simulink model "SS_design"  (R2025b)
settings: Solver=FixedStepAuto  StartTime=0.0  StopTime=0.0061  FixedStep=1/85e3/1500  RelTol=1e-3
values from neighbouring files (symbols this model uses):
  SS_DB = 0.01    [SS_topology_design.m]
  SS_Duty = 0.5    [SS_topology_design.m]
  SS_Freq = 85e3    (= 85000)    [SS_topology_design.m]
  SS_k = local_get_base_var('SS_k',  0.2)    [SS_find_R_for_power_260407.m]    (also in SS_sweep_R_for_power_260313.m; SS_topology_design.m = 0.2; matlab_workspace.mat = 0.2)
  SS_R = SS_R3    (= 31.23)    [SS_topology_design.m]
  SS_SoftStarting_slope = SS_Vin / SS_SoftStarting_TransientTime    (= 3250000)    [SS_topology_design.m]
  SS_SoftStarting_StartPwmTBCTR = SS_SoftStarting_slope * SS_SoftStarting_StartPwmTime    (= 32.5)    [SS_topology_design.m]
  SS_SoftStarting_StopPwmTBCTR = SS_SoftStarting_slope * SS_SoftStarting_StopPwmTime    (= 19500)    [SS_topology_design.m]
  SS_Vin = local_get_base_var('SS_Vin', 380)    [SS_find_R_for_power_260407.m]    (also in SS_sweep_R_for_power_260313.m; SS_topology_design.m = 650; matlab_workspace.mat = 380)
libraries: fl_lib x26, nesl_utility x25, ee_lib x14, simulink x2
settings Model: Creator=jibin  LastModifiedBy=jibin

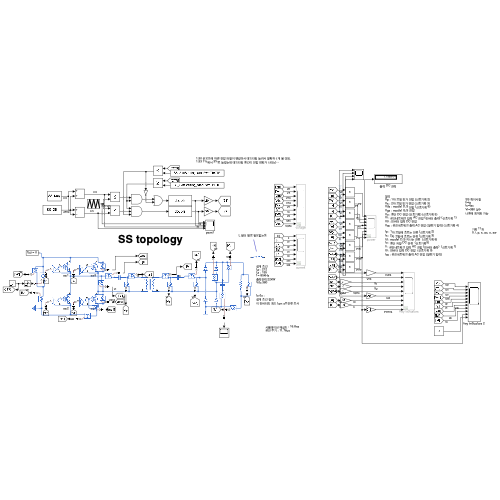
[thumbnail: Simulink's stored preview of the top-level diagram]
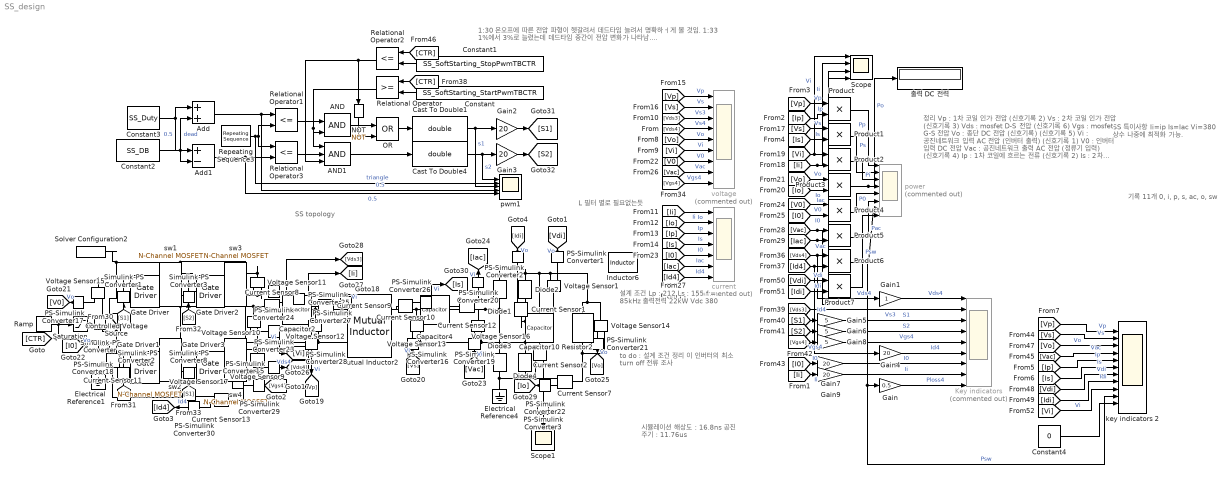
== system SS_design ==
  note: 시뮬레이션 해상도 : 16.8ns
      | 공진 주기 : 11.76us
  note: L 필터 별로 필요없는듯
  note: 기록 11개
      | 0, i, p, s, ac, o, sw
  note: SS 특이사항
      | Ii=ip
      | Is=Iac
      | Vi=380 상수
      | 나중에 최적화 가능.
  note: 정리
      | Vp : 1차 코일 인가 전압 (신호기록 2)
      | Vs : 2차 코일 인가 전압 (신호기록 3)
      | Vds : mosfet D-S 전압 (신호기록 6)
      | Vgs : mosfet G-S 전압
      | Vo : 종단 DC 전압 (신호기록) (신호기록 5)
      | Vi : 공진네트워크 입력 AC 전압 (인버터 출력) (신호기록 1)
      | V0 : 인버터 입력 DC 전압
      | Vac : 공진네트워크 출력 AC 전압 (정류기 입력) (신호기록 4)
      |
      | Ip : 1차 코일에 흐르는 전류 (신호기록 2)
      | Is : 2차 코일에 흐르는 전류 (신호기록 3)
      | Id : mosfet D-S 지나는 전류  (신호기록 6)
      | Io : 종단 저항 DC 전류  (신호기록5)
      | Ii : 공진네트워크 입력 AC 전압 (인버터 출력)  (신호기록 1)
      | I0 : 인버터 입력 DC 전압  (신호기록 0)
      | Iac : 공진네트워크 출력 AC 전압 (정류기 입력)
  note: 설계 조건
      | Lp : 212
      | Ls : 155
      | f = 85kHz
      | 출력전력 22kW
      | Vdc 380
  note: to do :
      | 설계 조건 정리
      | 이 인버터의 최소 turn off 전류 조사
  note: 1:30 온오프에 따른 전압 파형이 헷갈려서 데드타임 늘려서 명확하ㅓ게 볼 것임.
      | 1:33 1%에서 3%로 늘렸는데 데드타임 중간이 전압 변화가 나타남....
  note: SS topology
  AND : Logic  IconShape=distinctive  AllPortsSameDT=off  OutDataTypeStr=boolean
  AND1 : Logic  Inputs=3  IconShape=distinctive  AllPortsSameDT=off  OutDataTypeStr=boolean
  Add : Sum
  Add1 : Sum  Inputs=+-
  Capacitor10 : fl_lib/Electrical/Electrical Elements/Capacitor  c=SS_C_filter F  r=1e-6 Ohm  g=0 1/Ohm  i_specify=off  i_priority=None  i=0 A  i_nominal_specify=off  i_nominal_value=1  i_nominal_unit=A  v_specify=off  v_priority=None  v=0 V  v_nominal_specify=off  v_nominal_value=1  v_nominal_unit=V  vc_specify=off  vc_priority=High  vc=0 V  vc_nominal_specify=off  vc_nominal_value=1  vc_nominal_unit=V
  Capacitor2 : fl_lib/Electrical/Electrical Elements/Capacitor  c=SS_Cp F  r=1e-6 Ohm  g=0 1/Ohm  i_specify=off  i_priority=None  i=0 A  i_nominal_specify=off  i_nominal_value=1  i_nominal_unit=A  v_specify=off  v_priority=None  v=0 V  v_nominal_specify=off  v_nominal_value=1  v_nominal_unit=V  vc_specify=off  vc_priority=High  vc=0 V  vc_nominal_specify=off  vc_nominal_value=1  vc_nominal_unit=V
  Capacitor4 : fl_lib/Electrical/Electrical Elements/Capacitor  c=SS_Cs F  r=1e-6 Ohm  g=0 1/Ohm  i_specify=off  i_priority=None  i=0 A  i_nominal_specify=off  i_nominal_value=1  i_nominal_unit=A  v_specify=off  v_priority=None  v=0 V  v_nominal_specify=off  v_nominal_value=1  v_nominal_unit=V  vc_specify=off  vc_priority=High  vc=0 V  vc_nominal_specify=off  vc_nominal_value=1  vc_nominal_unit=V
  Cast To Double1 : DataTypeConversion  OutDataTypeStr=double  SaturateOnIntegerOverflow=off  RndMeth=Floor
  Cast To Double4 : DataTypeConversion  OutDataTypeStr=double  SaturateOnIntegerOverflow=off  RndMeth=Floor
  Constant : Constant  Value=SS_SoftStarting_StartPwmTBCTR
  Constant1 : Constant  Value=SS_SoftStarting_StopPwmTBCTR
  Constant2 : Constant  Value=SS_DB
  Constant3 : Constant  Value=SS_Duty
  Constant4 : Constant  Value=0
  Controlled Voltage Source : fl_lib/Electrical/Electrical Sources/Controlled Voltage Source
  Current Sensor{1..2,7..13} (9 alike) : fl_lib/Electrical/Electrical Sensors/Current Sensor
  Diode{1..4} (4 alike) : ee_lib/Semiconductors & Converters/Diode  ModelType=ee.enum.diode.modelType.pwl  TableType=ee.enum.diode.tableType.IfMat  IfMat=[.07, .12, .19, 1.75, 4.24, 7.32, 11.2; .16, .3, .72, 2.14, 5.02, 8.35, 13.12] A  VfMat=[.9, 1.15, 1.25, 1.5, 1.75, 2.17, 2.6, 2.85; .58, .68, .75, 1.1, 1.38, 1.77, 2.27, 2.7] V  TjVec=[25, 125] degC  VfVec=[.5, .7, .9, 1.3, 1.7, 2.1, 2.5] V  IfVec=[.1, .2, .5, 1, 2, 4, 7, 10] A  IrMat=[1e-06, 2e-06, 5e-06, 1e-05, 2.5e-05, 5e-05, .0001; 2e-06, 5e-06, 1e-05, 4e-05, 8e-05, .0002, .0005] A  VrMat=[10, 100, 200, 250, 300, 325, 350; 10, 70, 160, 220, 270, 300, 320] V  VrVec=[10, 20, 40, 50, 70, 80, 100] V  IrVec=[1e-06, 2e-06, 5e-06, 1e-05, 2e-05, 5e-05, .0001] A  Vf=1 V  Ron=0.02 Ohm  Goff=1e-8 S  prmExp=ee.enum.diode.expParam.useTwo  I12=[.0137, .545] A  V12=[.6, .7] V  RS=0 Ohm  Tmeas=298.15 K  IS=1e-12 A  ec=1  I1=0.0137 A  V1=0.6 V  N_series=1  N_parallel=2  ZenerEnable=false  Rz=0.3 Ohm  BV=inf V  C_param=ee.enum.diode.capParam.fixed  CJ=0 pF  CJ0=5 pF  Vvec=[.1, 10, 100] V  Cvec=[3.5, 1, .4] pF  VJ=1 V  Mgrad=0.5  FC=0.5  Q_param=ee.enum.diode.recoveryParam.off  iRM=-7.15 A  iF=4 A  didt=-750 A/us  trr_factor=3  trr=115 ns  Qrr=150 nA*s  Vr=-600 V  Ls=150 nH  Erec=0.03 J  TT=50 ns  tau=100 ns  T_param=ee.enum.diode.temperatureParam.off  Tdevice=298.15 K  I1_T2=0.245 A  V1_T2=0.5 V  IS_T2=1.25e-7 A  Tmeas2=125 degC  XTI_param=ee.enum.diode.xtiParam.pn  XTI=3  EG_param=ee.enum.diode.egapParam.material_si  EG=1.11 eV  dBVdT=0 V/K  enable_fault_input=simscape.enum.onoff.off  i_specify=off  i_priority=None  i=0 A  i_nominal_specify=off  i_nominal_value=1  i_nominal_unit=A  v_specify=off  v_priority=None  v=0 V  v_nominal_specify=off  v_nominal_value=1  v_nominal_unit=V  v_capacitor_specify=off  v_capacitor_priority=None  v_capacitor=0 V  v_capacitor_nominal_specify=off  v_capacitor_nominal_value=1  v_capacitor_nominal_unit=V  Qj_specify=off  Qj_priority=High  Qj=0 C  Qj_nominal_specify=off  Qj_nominal_value=1  Qj_nominal_unit=C  i_diode_specify=off  i_diode_priority=None  i_diode=0 A  i_diode_nominal_specify=off  i_diode_nominal_value=1  i_diode_nominal_unit=A  v_diode_specify=off  v_diode_priority=None  v_diode=0 V  v_diode_nominal_specify=off  v_diode_nominal_value=1  v_diode_nominal_unit=V  i_capacitor_specify=off  i_capacitor_priority=None  i_capacitor=0 A  i_capacitor_nominal_specify=off  i_capacitor_nominal_value=1  i_capacitor_nominal_unit=A  power_dissipated_specify=off  power_dissipated_priority=None  power_dissipated=0 W  power_dissipated_nominal_specify=off  power_dissipated_nominal_value=1  power_dissipated_nominal_unit=W  fidelity_level=ee.enum.diode.fidelity.includeChargeDyn  rec_loss_model=ee.enum.diode.reverseRecoveryModel.fixed  ErecVal=0 J  scaleWithIandV=true  ErecMat=zeros(2, 3) J  TjrecVec=[298.15, 398.15] K  IfrecVec=[.1, 1, 10] A  IrecVal=10 A  VrecVal=10 V  tFilter=1 / 1000 / 100 s  thermal_network_parameterization=ee.enum.thermalNetworkTopology.junctionCase  Rth=[0, 10] K/W  Rth_Cauer=[1, 3, 10] K/W  Rth_Foster=[.08, .14, .22, .16] K/W  thermal_mass_parameterization=ee.enum.thermalNetwork.timeconstant  thermal_mass=[0, 1] J/K  thermal_mass_Cauer=[.1, .3, 1] J/K  thermal_mass_Foster=[.001, .005, .05, .5] J/K  thermal_time_constant=[0, 10] s  thermal_time_constant_Cauer=[1, 3, 10] s  thermal_time_constant_Foster=[7e-05, .0007, .01, .08] s  thermal_mass_initial_temperatures=[25, 25] degC  thermal_mass_initial_temperatures_Cauer=[25, 25, 25] degC  junction_thermal_mass=0.01 J/K  Tvec_initial_Foster=[25, 25, 25, 25] degC  no_thermal_network=0  junction_temperature_specify=off  junction_temperature_priority=None  junction_temperature=25 degC  junction_temperature_nominal_specify=off  junction_temperature_nominal_value=1  junction_temperature_nominal_unit=degC
  Electrical Reference1 : fl_lib/Electrical/Electrical Elements/Electrical Reference
  Electrical Reference4 : fl_lib/Electrical/Electrical Elements/Electrical Reference
  Gain : Gain  Gain=0.5
  Gain1 : Gain
  Gain{2..4,7,9} (5 alike) : Gain  Gain=20
  Gain5 : Gain  Gain=5
  Gain6 : Gain  Gain=5
  Gain8 : Gain  Gain=5
  Gate Driver{,1..3} (4 alike) : ee_lib/Semiconductors & Converters/Gate Driver  port_option=ee.enum.controlport.ps  uHigh=2.0 V  uLow=0.8 V  uHighValue=0.7  uLowValue=0.3  vHigh=SS_driv_Von V  vLow=SS_driv_Voff V  tHigh=0 ns  tLow=0 ns  parameterization=ee.enum.semiconductors.gateDriverParam.outputImpedance  rHigh=15 Ohm  rLow=15 Ohm  tRise=20 ns  tFall=20 ns  cLoad=10 nF  ZonTime_specify=off  ZonTime_priority=None  ZonTime=0 s  ZoffTime_specify=off  ZoffTime_priority=None  ZoffTime=0 s
      settings: InternalSimscapePortConfiguration="{\"Bottom\":[],\"Left\":[{\"id\":\"u\",\"label\":\"u\",\"type\":\"input\"}],\"Right\":[{\"id\":\"G\",\"label\":\"G\",\"type\":\"foundation.electrical.electrical\"},{\"id\":\"S\",\"label\":\"S\",\"type\":\"foundation.electrical.electrical\"}],\"Top\":[]}"
  Inductor6 : ee_lib/Passive/Inductor  l=SS_L_filter H  enable_L_tol=ee.enum.toleranceApplication.none  L_tol=20  tol_distribution=ee.enum.toleranceDistribution.uniform  nSigma=4  r=0 Ohm  g=1e-9 1/Ohm  enable_operating_limits=ee.enum.enable.no  operating_limit_action=ee.enum.passive.reportOpLim.warn  max_working_current=1 A  power_rating=1 W  i_L_specify=off  i_L_priority=High  i_L=0 A  i_L_nominal_specify=off  i_L_nominal_value=1  i_L_nominal_unit=A
  Key indicators : Scope  Commented=on  NumInputPorts=9
      settings: ActiveDisplayYMinimum=-3153.8043983257576  ActiveDisplayYMaximum=2006.1519840284409  DataLoggingVariableName=ScopeData3
  Mutual Inductor2 : ee_lib/Passive/Transformers/Mutual Inductor  L1=SS_Lp H  L2=SS_Ls H  k=SS_k  L_tol=0  enable_L1_tol=ee.enum.toleranceApplication.none  L1_tol_distribution=ee.enum.toleranceDistribution.uniform  L1_nSigma=4  enable_L2_tol=ee.enum.toleranceApplication.none  L2_tol_distribution=ee.enum.toleranceDistribution.uniform  L2_nSigma=4  r=[.001, .001] Ohm  g=[1e-09, 1e-09] 1/Ohm  enable_operating_limits=ee.enum.enable.no  operating_limit_action=ee.enum.passive.reportOpLim.warn  max_working_current=1 A  power_rating=1 W  iL1_specify=off  iL1_priority=High  iL1=0 A  iL1_nominal_specify=off  iL1_nominal_value=1  iL1_nominal_unit=A  iL2_specify=off  iL2_priority=High  iL2=0 A  iL2_nominal_specify=off  iL2_nominal_value=1  iL2_nominal_unit=A
      settings: InternalSimscapePortConfiguration="{\"Bottom\":[],\"Left\":[{\"id\":\"p1\",\"label\":\"1+\",\"type\":\"foundation.electrical.electrical\"},{\"id\":\"n1\",\"label\":\"1-\",\"type\":\"foundation.electrical.electrical\"}],\"Right\":[{\"id\":\"p2\",\"label\":\"2+\",\"type\":\"foundation.electrical.electrical\"},{\"id\":\"n2\",\"label\":\"2-\",\"type\":\"foundation.electrical.electrical\"}],\"Top\":[]}"
  NOT : Logic  Operator=NOT  IconShape=distinctive  AllPortsSameDT=off  OutDataTypeStr=boolean
  OR : Logic  Operator=OR  IconShape=distinctive  AllPortsSameDT=off  OutDataTypeStr=boolean
  PS-Simulink Converter{1..3,15..30} (19 alike) : nesl_utility/PS-Simulink Converter  PhysicalDomain=network_engine_domain  SubClassName=ps_output  LeftPortType=input  RightPortType=output  PseudoPeriodic=off  Frequencies=[]  VectorFormat=inherit  Unit=inherit  AffineConversion=off
  Product{,1..7} (8 alike) : Product
  Ramp : simulink/Sources/Ramp  slope=SS_SoftStarting_slope  start=SS_SoftStarting_delayed  InitialOutput=0
  Relational Operator : RelationalOperator  OutDataTypeStr=boolean  RndMeth=Simplest  InputSameDT=off
  Relational Operator1 : RelationalOperator  Operator=<=  OutDataTypeStr=boolean  RndMeth=Simplest  InputSameDT=off
  Relational Operator2 : RelationalOperator  Operator=<=  OutDataTypeStr=boolean  RndMeth=Simplest  InputSameDT=off
  Relational Operator3 : RelationalOperator  Operator=<=  OutDataTypeStr=boolean  RndMeth=Simplest  InputSameDT=off
  Repeating Sequence3 : simulink/Sources/Repeating Sequence  rep_seq_t=[0 1/SS_Freq/2 1/SS_Freq]  rep_seq_y=[0 1 0]
  Resistor2 : fl_lib/Electrical/Electrical Elements/Resistor  R=SS_R Ohm  i_specify=off  i_priority=None  i=0 A  i_nominal_specify=off  i_nominal_value=1  i_nominal_unit=A  v_specify=off  v_priority=None  v=0 V  v_nominal_specify=off  v_nominal_value=1  v_nominal_unit=V
  Saturation : Saturate  UpperLimit=SS_Vin  LowerLimit=0
  Scope : Scope  NumInputPorts=4
      settings: ActiveDisplayYMinimum=-209.64709270846973  ActiveDisplayYMaximum=229.34788450491459  DataLoggingVariableName=ScopeData6
  Scope1 : Scope
      settings: ActiveDisplayYMinimum=-22.784253900925922  ActiveDisplayYMaximum=48.876040057618852  DataLoggingVariableName=ScopeData7
  Simulink-PS Converter{,1..3,8} (5 alike) : nesl_utility/Simulink-PS Converter  PhysicalDomain=network_engine_domain  SubClassName=ps_input  LeftPortType=input  RightPortType=output  PseudoPeriodic=off  Frequencies=[]  NoiseDistribution=none  NoiseParameters=[]  Unit=1  AffineConversion=off  FilteringAndDerivatives=provide  SimscapeFilterOrder=1  InputFilterTimeConstant=0.001  UdotUserProvided=0
  Solver Configuration2 : nesl_utility/Solver Configuration  PhysicalDomain=network_engine_domain  SubClassName=solver  LeftPortType=input  RightPortType=generic  Tones=[]  Harmonics=[]  SimulateNoise=off  Profile=off  UseLocalSampling=off  EnableSwitchedLinearOptims=on  FrequencyDomain=off  UseCCode=off  RelTol=0.001  AbsTol=0.001  MinStep=1e-09  ToWorkspace=off  RevertToSquareIcSolve=off  NumHomotopyIterations=100  PhasorMode=off  PhasorModeNumHarmonics=1  ConsistencySolver=NEWTON_XTOL_AFTER_FTOL  IndexReductionMethod=DerivativeReplacement  DoDC=off  ResidualTolerance=1e-09  ConsistencyTolSource=LOCAL  ConsistencyAbsTol=0.001  ConsistencyRelTol=0.001  ConsistencyTolFactor=0.001  UseLocalSolver=on  LocalSolverChoice=NE_BACKWARD_EULER_ADVANCER  ResolveIndetEquations=on  FunctionEvalNumThread=1  LocalSolverSampleTime=1/85e3/1500  DoFixedCost=off  MaxNonlinIter=3  MaxModeIter=2  ComputeImpulses=off  ImpulseIterations=2  LinearAlgebra=auto  LinearAlgebraNumThread=0  EquationFormulation=NE_TIME_EF  DelaysMemoryBudget=1024  AutomaticFiltering=on  FilteringTimeConstant=0.001  PartitionStorageMethod=AS_NEEDED  PartitionMemoryBudget=1024  PartitionMethod=ROBUST  MultibodyUseLocalSolver=off  MultibodyLocalSolverChoice=ODE1  MultibodyLocalSolverSampleTime=0.001
  Voltage Sensor{1,9..17} (10 alike) : fl_lib/Electrical/Electrical Sensors/Voltage Sensor
  current : Scope  Commented=on  NumInputPorts=7
      settings: ActiveDisplayYMinimum=-15.036920895804315  ActiveDisplayYMaximum=15.036548168459881  DataLoggingVariableName=ScopeData5
  key indicators 2 : Scope  NumInputPorts=11
      settings: ActiveDisplayYMinimum=-48.81005828333268  ActiveDisplayYMaximum=48.809899474226675  DataLoggingVariableName=ScopeData4
  power : Scope  Commented=on  NumInputPorts=8
      settings: ActiveDisplayYMinimum=-2917.4741036570072  ActiveDisplayYMaximum=7376.975692043733
  pwm1 : Scope  NumInputPorts=5
      settings: ActiveDisplayYMinimum=-0.12497287522603978  ActiveDisplayYMaximum=1.1247558770343582
  sw{1..4} (4 alike) : ee_lib/Semiconductors & Converters/N-Channel MOSFET  paramTerminal=ee.enum.mosfet.numberOfTerminals.three  parameterization=ee.enum.mosfet.parameterization.datasheet  Beta=5.0 A/V^2  Rds=15 mOhm  Id=100 A  Vgs=15 V  Vth=2.5 V  Vth0=1.7 V  lam=0 1/V  gamma_vth=0.5 V^(1/2)  phib=0.5 V  Vth1=1.9071 V  Vbs1=-1 V  Vth2=2.066 V  Vbs2=-2 V  Tmeas=25 degC  Vgs_vec=[-1, -.5, 2, 3, 4, 5] V  Vds_vec=[0, 2, 4, 8, 12, 16, 20] V  Vbs_vec=[0, -4, -6, -12] V  T_vec=[25, 125] degC  Vth_vec=[.4, 1.2, 1.4, 1.45] V  Vth_mat=[.4, .35; 1.2, 1.15; 1.4, 1.35; 1.45, 1.4] V  Ids_mat=[0, 0, 0, 0, 0, 0, 0; 0, 0, 0, 0, 0, 0, 0; 0, .003, .0038, .0043, .0046, .0048, .0049; 0, .0055, .008, .009, .0095, .01, .0101; 0, .0115, .016, .018, .019, .0195, .02; 0, .0152, .0225, .0265, .028, .0295, .03] A  Ids_mat0=[0, 0, 0, 0, 0, 0, 0; 0, 0, 0, 0, 0, 0, 0; 0, .003, .0038, .0043, .0046, .0048, .0049; 0, .0055, .008, .009, .0095, .01, .0101; 0, .0115, .016, .018, .019, .0195, .02; 0, .0152, .0225, .0265, .028, .0295, .03] A  Ids_mat_3D=zeros(6, 7, 2) A  Ids_mat_3D0=zeros(6, 7, 2) A  IV_table_symmetry=ee.enum.mosfet.symmetricNIV.no  RS=0.0001 Ohm  RD=0.01 Ohm  RB=0.001 Ohm  LeadRs=1e-4 Ohm  LeadRd=1e-4 Ohm  LeadRg=1e-4 Ohm  LeadRb=0 Ohm  LS=1e-4 nH  LD=1e-4 nH  LG=1e-4 nH  LB=0 nH  C_param=ee.enum.mosfet.capacitanceParam.fixedciss  C_GS=270 pF  C_GD=80 pF  C_GB=0 pF  C_DS=0 pF  C_iss=SS_MSFT_Ciss F  C_rss=SS_MSFT_Crss F  C_oss=SS_MSFT_Coss F  C_iss_vec=[720, 700, 590, 470, 390, 310] pF  C_rss_vec=[450, 400, 300, 190, 95, 55] pF  C_oss_vec=[900, 810, 690, 420, 270, 170] pF  C_GS_vec=[270, 300, 290, 280, 295, 255] pF  C_GD_vec=[450, 400, 300, 190, 95, 55] pF  C_GB_vec=[270, 300, 290, 280, 295, 255] pF  C_Vgs_vec=0 V  C_DS_vec=[450, 410, 390, 230, 175, 115] pF  C_Vds_vec=[.1, .3, 1, 3, 10, 30] V  V_GS_for_cap_data=0 V  charge_linearity_param=ee.enum.mosfet.cgdLinearity.constant  C_OX=200 pF  V_C_OX=-0.5 V  charge_linearity_param_vgb=ee.enum.mosfet.cgbLinearity.instantly  charge_linearity_param_with_vgb=ee.enum.mosfet.cgbLinearityWithSeparateCgb.instantly  Di_param=ee.enum.mosfet.diodeParam.exponential  IsDiode=1e-12 A  Vbi=0.6 V  n=1  Cj0Diode=0 pF  TT=150e-9 s  Tmeas_dio=25 degC  TableTypeNoT=ee.enum.mosfet.tableType.IfMat  TableType=ee.enum.diode.tableType.IfMat  IfVec=[.07, .12, .19, 1.75, 4.24, 7.32, 11.2] A  IfMat=[.07, .12, .19, 1.75, 4.24, 7.32, 11.2; .16, .3, .72, 2.14, 4.02, 6.35, 9.12] A  VfVecV=[.9, 1.15, 1.25, 1.5, 1.75, 2.17, 2.6, 2.85] V  VfMatV=[.9, 1.15, 1.25, 1.5, 1.75, 2.17, 2.6, 2.85; .58, .68, .75, 1.1, 1.38, 1.77, 2.27, 2.7] V  TjVec=[25, 125] degC  VfVec=[.5, .7, .9, 1.3, 1.7, 2.1, 2.5] V  IfVecV=[.1, .2, .5, 1, 2, 4, 7, 10] A  diode_Goff=1e-12 1/Ohm  prmDatasheet=ee.enum.temperatureParameterization.none  prmEquCoeff=ee.enum.temperatureParameterization.none  dVth_dT=-6 mV/K  dVth0_dT=-6 mV/K  Rds_T2=0.037 Ohm  BEXDatasheet=-1.5  BEXEquCoeff=-1.5  etaisDatasheet=3  etaisEquCoeff=3  Tmeas2=125 degC  etaisTabulated=3  TdeviceDatasheet=25 degC  TdeviceEquCoeff=25 degC  TdeviceTabulated=25 degC  i_g_specify=off  i_g_priority=None  i_g=0 A  i_g_nominal_specify=off  i_g_nominal_value=1  i_g_nominal_unit=A  i_d_specify=off  i_d_priority=None  i_d=0 A  i_d_nominal_specify=off  i_d_nominal_value=1  i_d_nominal_unit=A  i_b_specify=off  i_b_priority=None  i_b=0 A  i_b_nominal_specify=off  i_b_nominal_value=1  i_b_nominal_unit=A  voltage_gs_specify=off  voltage_gs_priority=None  voltage_gs=0 V  voltage_gs_nominal_specify=off  voltage_gs_nominal_value=1  voltage_gs_nominal_unit=V  voltage_ds_specify=off  voltage_ds_priority=None  voltage_ds=0 V  voltage_ds_nominal_specify=off  voltage_ds_nominal_value=1  voltage_ds_nominal_unit=V  voltage_bs_specify=off  voltage_bs_priority=None  voltage_bs=0 V  voltage_bs_nominal_specify=off  voltage_bs_nominal_value=1  voltage_bs_nominal_unit=V  v_Cgs_specify=on  v_Cgs_priority=None  v_Cgs=0 V  v_Cgs_nominal_specify=off  v_Cgs_nominal_value=1  v_Cgs_nominal_unit=V  v_Cds_specify=on  v_Cds_priority=None  v_Cds=0 V  v_Cds_nominal_specify=off  v_Cds_nominal_value=1  v_Cds_nominal_unit=V  v_Cbs_specify=off  v_Cbs_priority=High  v_Cbs=0 V  v_Cbs_nominal_specify=off  v_Cbs_nominal_value=1  v_Cbs_nominal_unit=V  thermal_network_parameterization=ee.enum.thermalNetworkTopology.junctionCase  Rth=[0, 10] K/W  Rth_Cauer=[1, 3, 10] K/W  Rth_Foster=[.08, .14, .22, .16] K/W  thermal_mass_parameterization=ee.enum.thermalNetwork.timeconstant  thermal_mass=[0, 1] J/K  thermal_mass_Cauer=[.1, .3, 1] J/K  thermal_mass_Foster=[.001, .005, .05, .5] J/K  thermal_time_constant=[0, 10] s  thermal_time_constant_Cauer=[1, 3, 10] s  thermal_time_constant_Foster=[7e-05, .0007, .01, .08] s  thermal_mass_initial_temperatures=[25, 25] degC  thermal_mass_initial_temperatures_Cauer=[25, 25, 25] degC  Tvec_initial_Foster=[25, 25, 25, 25] degC  betaref=18 A/V^2  Vfbref=-1.1 V  gamma=3.5 V^(1/2)  phib2ref=1 V  thesatref=0.4 1/V  alpha=0  Vp=5e-2 V  thesrref=0 1/V  m=8  Tref=25 degC  Rsref=2e-3 Ohm  Rdref=0.17 Ohm  Rgref=8.4 Ohm  Rbref=2e-3 Ohm  Cox=1500 pF  Cgso=100 pF  Cgdo=14 pF  Isref=5.2e-13 A  Cj0=480 pF  Tprm=1  etabet=1.3  Stvfb=5e-4 V/K  Stphib=-8.5e-4 V/K  etasat=1.04  etasr=0.65  etar=0.95  etais=3  Tsim=25 degC  Ig_specify=off  Ig_priority=None  Ig=0 A  Ig_nominal_specify=off  Ig_nominal_value=1  Ig_nominal_unit=nA  Ids_specify=off  Ids_priority=None  Ids=0 A  Ids_nominal_specify=off  Ids_nominal_value=1  Ids_nominal_unit=A  Ib_specify=off  Ib_priority=None  Ib=0 A  Ib_nominal_specify=off  Ib_nominal_value=1  Ib_nominal_unit=uA  V_gs_specify=off  V_gs_priority=None  V_gs=0 V  V_gs_nominal_specify=off  V_gs_nominal_value=1  V_gs_nominal_unit=V  V_ds_specify=off  V_ds_priority=None  V_ds=0 V  V_ds_nominal_specify=off  V_ds_nominal_value=1  V_ds_nominal_unit=V  V_bs_specify=off  V_bs_priority=None  V_bs=0 V  V_bs_nominal_specify=off  V_bs_nominal_value=1  V_bs_nominal_unit=V  QGoverCox_specify=off  QGoverCox_priority=None  QGoverCox=0 V  QGoverCox_nominal_specify=off  QGoverCox_nominal_value=1  QGoverCox_nominal_unit=V  QDoverCox_specify=off  QDoverCox_priority=None  QDoverCox=0 V  QDoverCox_nominal_specify=off  QDoverCox_nominal_value=1  QDoverCox_nominal_unit=V  QBoverCox_specify=off  QBoverCox_priority=None  QBoverCox=0 V  QBoverCox_nominal_specify=off  QBoverCox_nominal_value=1  QBoverCox_nominal_unit=V  T0=[25, 25] degC  T0_Cauer=[25, 25, 25] degC
  voltage : Scope  Commented=on  NumInputPorts=9
      settings: ActiveDisplayYMinimum=-88.829095611503391  ActiveDisplayYMaximum=432.28140472052308  DataLoggingVariableName=ScopeData2
  출력 DC 전력 : Display
  wires:
  Product6/1 -> key indicators 2/10, Gain/1, power/7  "Psw"
  Add1/1 -> pwm1/5, Relational Operator3/2  "0.5"
  [Vds4] -> voltage/4  "Vs4"
  [Io] -> current/2  "Io"
  Product4/1 -> power/5  "P0"
  Product/1 -> power/1  "Pp"
  [I0] -> current/5  "I0"
  Relational Operator3/1 -> AND1/2
  Gain5/1 -> Key indicators/3  "S1"
  PS-Simulink Converter25/1 -> [Ii]
  OR/1 -> Cast To Double1/1
  [Ii] -> Scope/2, Product2/2  "Ii"
  [Vi] -> voltage/6  "Vi"
  PS-Simulink Converter29/1 -> [Vgs4]
  PS-Simulink Converter26/1 -> [Is]  "Vi"
  [Iac] -> Scope/4, Product5/2  "Iac"
  [S2] -> Simulink-PS Converter3/1
  Product2/1 -> power/3  "Pi"
  Gain1/1 -> Key indicators/1  "Vds4"
  [S1] -> Simulink-PS Converter1/1
  Relational Operator1/1 -> AND/1
  [CTR] -> Relational Operator2/1
  [Vi] -> Scope/1, Product2/1  "Vi"
  AND/1 -> OR/1
  Constant2/1 -> Add/2, Add1/2  "dead"
  Cast To Double1/1 -> Gain2/1, pwm1/3  "s1"
  [CTR] -> Relational Operator/1
  [Ip] -> current/3  "Ip"
  [Ip] -> Product/2  "Ip"
  NOT/1 -> OR/2
  [Vs] -> Product1/1  "Vs"
  Gain8/1 -> Key indicators/5  "Vgs4"
  [Id4] -> Gain4/1, Product6/2  "Id4"
  Relational Operator/1 -> AND1/1, AND/2
  Product5/1 -> power/6  "Pac"
  Constant3/1 -> Add/1, Add1/1  "0.5"
  [V0] -> Product4/1  "V0"
  Cast To Double4/1 -> Gain3/1, pwm1/1  "s2"
  Gain2/1 -> [S1]
  [Vo] -> voltage/5  "Vo"
  [Vac] -> voltage/8  "Vac"
  [S1] -> Simulink-PS Converter8/1
  [Io] -> Product3/2  "Io"
  Gain4/1 -> Key indicators/6  "Id4"
  PS-Simulink Converter19/1 -> [Vac]  "Vi"
  PS-Simulink Converter30/1 -> [Id4]  "Id4"
  [Id4] -> current/7  "Id4"
  [Vgs4] -> Gain8/1  "Vgs4"
  [S2] -> Simulink-PS Converter2/1
  [Vo] -> Product3/1  "Vo"
  PS-Simulink Converter21/1 -> [Vo]  "Vo"
  PS-Simulink Converter17/1 -> [V0]  "Vo"
  Repeating Sequence3/1 -> pwm1/2, Relational Operator1/2, Relational Operator3/1  "triangle"
  [S2] -> Gain6/1
  [Vac] -> Scope/3, Product5/1  "Vac"
  PS-Simulink Converter22/1 -> [Io]
  Gain6/1 -> Key indicators/4  "S2"
  Saturation/1 -> Simulink-PS Converter/1
  PS-Simulink Converter18/1 -> [I0]  "Vo"
  Product1/1 -> power/2  "Ps"
  Ramp/1 -> Saturation/1, [CTR]
  [Vp] -> Product/1  "Vp"
  PS-Simulink Converter27/1 -> [Ip]  "Vi"
  [Vds3] -> Key indicators/2  "Vs3"
  Gain3/1 -> [S2]
  Gain7/1 -> Key indicators/7  "I0"
  PS-Simulink Converter16/1 -> [Vs]  "Vi"
  [Vds3] -> voltage/3  "Vs3"
  AND1/1 -> Cast To Double4/1
  PS-Simulink Converter20/1 -> [Iac]  "Vi"
  Constant/1 -> Relational Operator/2
  PS-Simulink Converter24/1 -> [Vds3]
  [Vgs4] -> voltage/9  "Vgs4"
  [I0] -> Product4/2  "I0"
  Product3/1 -> 출력 DC 전력/1, power/4  "Po"
  PS-Simulink Converter28/1 -> [Vp]  "Vi"
  [Is] -> Product1/2  "Is"
  [S1] -> Gain5/1
  [Ii] -> current/1  "Ii"
  [V0] -> voltage/7  "V0"
  [I0] -> Gain7/1  "I0"
  [Vs] -> voltage/2  "Vs"
  Relational Operator2/1 -> NOT/1, AND1/3
  [Iac] -> current/6  "Iac"
  Gain/1 -> Key indicators/9  "Ploss4"
  [Vp] -> voltage/1  "Vp"
  Constant1/1 -> Relational Operator2/2
  PS-Simulink Converter23/1 -> [Vi]  "Vi"
  [Vds4] -> Gain1/1, Product6/1  "Vds4"
  PS-Simulink Converter15/1 -> [Vds4]  "Vds4"
  Add/1 -> pwm1/4, Relational Operator1/1  "0.5"
  [Is] -> current/4  "Is"
  [Ii] -> Gain9/1  "Ii"
  Gain9/1 -> Key indicators/8  "Ii"
  [Vp] -> key indicators 2/1  "Vp"
  [Vs] -> key indicators 2/2  "Vs"
  [Vo] -> key indicators 2/3  "Vo"
  [Vac] -> key indicators 2/4  "Vac"
  [Ip] -> key indicators 2/5  "Ip"
  [Is] -> key indicators 2/6  "Is"
  PS-Simulink Converter1/1 -> [Vdi]  "Vo"
  [Vdi] -> key indicators 2/7  "Vdi"
  [Idi] -> key indicators 2/8  "Idi"
  PS-Simulink Converter2/1 -> [Idi]  "Vo"
  [Vdi] -> Product7/1  "Vdi"
  [Idi] -> Product7/2  "Idi"
  Product7/1 -> power/8  "Psw"
  [Vi] -> key indicators 2/9  "Vi"
  Constant4/1 -> key indicators 2/11
  PS-Simulink Converter3/1 -> Scope1/1
  connections:
  Voltage Sensor10/RConn2 -- Voltage Sensor12/RConn2 -- Mutual Inductor2/LConn2 -- Voltage Sensor9/LConn1 -- sw4/RConn1 -- Voltage Sensor11/RConn2 -- sw3/RConn2 -- Gate Driver2/RConn2
  Diode4/LConn1 -- Diode3/LConn1 -- Electrical Reference4/LConn1 -- Current Sensor2/RConn2 -- Current Sensor7/RConn2
  Gate Driver/RConn2 -- sw1/RConn2 -- Current Sensor8/LConn1 -- Voltage Sensor10/LConn1 -- sw2/RConn1
  Gate Driver3/RConn1 -- sw4/LConn1 -- Voltage Sensor17/LConn1
  Gate Driver3/RConn2 -- Voltage Sensor9/RConn2 -- sw4/RConn2 -- Current Sensor13/LConn1 -- Voltage Sensor17/RConn2
  Voltage Sensor15/RConn2 -- Current Sensor11/RConn2 -- Controlled Voltage Source/RConn2
  sw2/RConn2 -- Gate Driver1/RConn2 -- Electrical Reference1/LConn1 -- Current Sensor11/LConn1 -- Current Sensor13/RConn2
  Resistor2/RConn1 -- Current Sensor7/LConn1 -- Voltage Sensor14/RConn2
  sw1/RConn1 -- Controlled Voltage Source/LConn1 -- Voltage Sensor15/LConn1 -- Solver Configuration2/RConn1 -- Voltage Sensor11/LConn1 -- sw3/RConn1
  Capacitor10/LConn1 -- Diode2/RConn1 -- Diode1/RConn1 -- Resistor2/LConn1 -- Voltage Sensor14/LConn1 -- Voltage Sensor1/RConn2
  Mutual Inductor2/RConn2 -- Diode4/RConn1 -- Current Sensor1/LConn1 -- Voltage Sensor1/LConn1 -- Voltage Sensor16/RConn2 -- Voltage Sensor13/RConn2
  Capacitor2/RConn1 -- Current Sensor9/LConn1 -- Voltage Sensor12/LConn1
  Capacitor4/LConn1 -- Voltage Sensor13/LConn1 -- Current Sensor10/RConn2
  Current Sensor12/RConn2 -- Voltage Sensor16/LConn1 -- Diode3/RConn1 -- Diode1/LConn1
  PS-Simulink Converter17/LConn1 -- Voltage Sensor15/RConn1
  PS-Simulink Converter27/LConn1 -- Current Sensor9/RConn1
  Voltage Sensor16/RConn1 -- PS-Simulink Converter19/LConn1
  Current Sensor7/RConn1 -- PS-Simulink Converter22/LConn1
  Simulink-PS Converter2/RConn1 -- Gate Driver1/LConn1
  Gate Driver3/LConn1 -- Simulink-PS Converter8/RConn1
  Simulink-PS Converter1/RConn1 -- Gate Driver/LConn1
  PS-Simulink Converter20/LConn1 -- Current Sensor12/RConn1
  sw3/LConn1 -- Gate Driver2/RConn1
  PS-Simulink Converter21/LConn1 -- Voltage Sensor14/RConn1
  Current Sensor13/RConn1 -- PS-Simulink Converter30/LConn1
  Gate Driver1/RConn1 -- sw2/LConn1
  Simulink-PS Converter3/RConn1 -- Gate Driver2/LConn1
  PS-Simulink Converter18/LConn1 -- Current Sensor11/RConn1
  Current Sensor9/RConn2 -- Mutual Inductor2/LConn1
  PS-Simulink Converter25/LConn1 -- Current Sensor8/RConn1
  Mutual Inductor2/RConn1 -- Current Sensor10/LConn1
  Capacitor2/LConn1 -- Current Sensor8/RConn2
  Voltage Sensor12/RConn1 -- PS-Simulink Converter28/LConn1
  Voltage Sensor13/RConn1 -- PS-Simulink Converter16/LConn1
  PS-Simulink Converter24/LConn1 -- Voltage Sensor11/RConn1
  PS-Simulink Converter15/LConn1 -- Voltage Sensor9/RConn1
  PS-Simulink Converter29/LConn1 -- Voltage Sensor17/RConn1
  sw1/LConn1 -- Gate Driver/RConn1
  Simulink-PS Converter/RConn1 -- Controlled Voltage Source/RConn1
  PS-Simulink Converter23/LConn1 -- Voltage Sensor10/RConn1
  Current Sensor10/RConn1 -- PS-Simulink Converter26/LConn1
  Capacitor4/RConn1 -- Current Sensor12/LConn1
  PS-Simulink Converter1/LConn1 -- Voltage Sensor1/RConn1
  Diode2/LConn1 -- Current Sensor1/RConn2
  Current Sensor1/RConn1 -- PS-Simulink Converter2/LConn1
  Current Sensor2/LConn1 -- Capacitor10/RConn1
  PS-Simulink Converter3/LConn1 -- Current Sensor2/RConn1
